simulink model "Pokus02_3bit_Counter"  (Simulink 8.1)
settings: Solver=ode45  StartTime=0.0  StopTime=20  RelTol=1e-3
undefined symbols (not defined in the file): sigbuilder_block
libraries: simulink_extras x17, Common_Library x9, commutil2 x4
settings Model: Creator=uzivatel  LastModifiedBy=uzivatel
settings DataIOCC: SignalLoggingSaveFormat=Dataset
settings OptimizationCC: ExpressionDepthLimit=128
settings DebuggingCC: FcnCallInpInsideContextMsg=EnableAllAsError
settings GRTTargetCC: CombineOutputUpdateFcns=on  GRTInterface=off

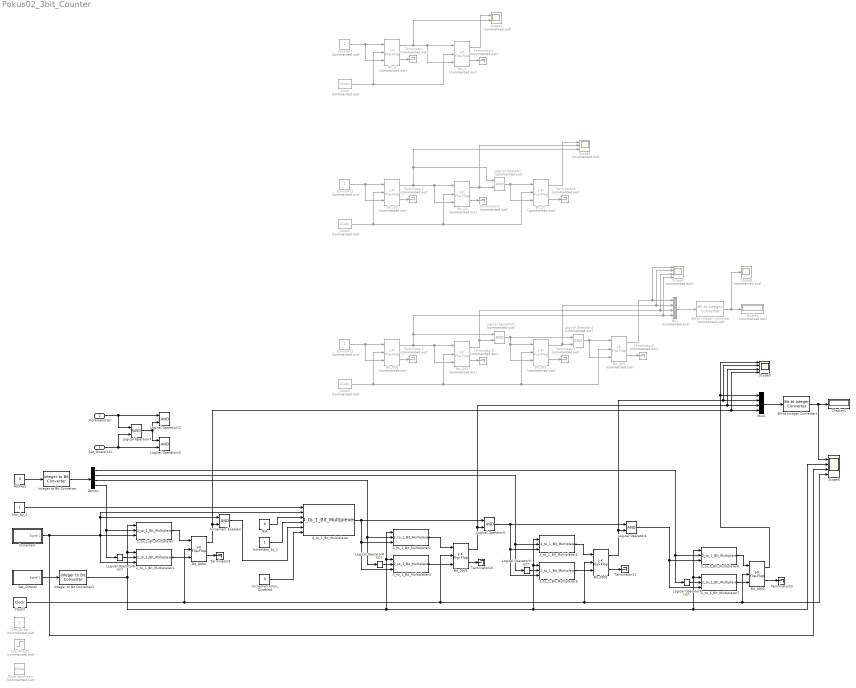
== system Pokus02_3bit_Counter ==
  Set_Direct(1b) : Inport
  Increment(1b) : Inport  Port=2
  2_to_1_Bit_Multiplexer{,1..7} (8 alike) : Common_Library/Multiplexers/2_to_1_Bit_Multiplexer
  4_to_1_Bit_Multiplexer : Common_Library/Multiplexers/4_to_1_Bit_Multiplexer
  Address : Constant  Value=3  OutDataTypeStr=uint8
  Bit to Integer Converter : commutil2/Bit to Integer Converter  Commented=on  nbits=4  bitOrder=MSB first  signedOutputValues=Unsigned  outDtype=uint8  outDtypeSigned=Inherit via internal rule
  Bit to Integer Converter1 : commutil2/Bit to Integer Converter  nbits=4  bitOrder=MSB first  signedOutputValues=Unsigned  outDtype=uint8  outDtypeSigned=Inherit via internal rule
  Bit_0 : simulink_extras/Flip Flops/J-K Flip-Flop  Commented=on  initial_condition=0
  Bit_00 : simulink_extras/Flip Flops/J-K Flip-Flop  Commented=on  initial_condition=0
  Bit_000 : simulink_extras/Flip Flops/J-K Flip-Flop  Commented=on  initial_condition=0
  Bit_0000 : simulink_extras/Flip Flops/J-K Flip-Flop  initial_condition=0
  Bit_0001 : simulink_extras/Flip Flops/J-K Flip-Flop  initial_condition=0
  Bit_0002 : simulink_extras/Flip Flops/J-K Flip-Flop  initial_condition=0
  Bit_0003 : simulink_extras/Flip Flops/J-K Flip-Flop  initial_condition=0
  Bit_001 : simulink_extras/Flip Flops/J-K Flip-Flop  Commented=on  initial_condition=0
  Bit_002 : simulink_extras/Flip Flops/J-K Flip-Flop  Commented=on  initial_condition=0
  Bit_003 : simulink_extras/Flip Flops/J-K Flip-Flop  Commented=on  initial_condition=0
  Bit_01 : simulink_extras/Flip Flops/J-K Flip-Flop  Commented=on  initial_condition=0
  Bit_02 : simulink_extras/Flip Flops/J-K Flip-Flop  Commented=on  initial_condition=0
  Bit_1 : simulink_extras/Flip Flops/J-K Flip-Flop  Commented=on  initial_condition=0
  Clock : simulink_extras/Flip Flops/Clock  Commented=on  period=1
  Clock1 : simulink_extras/Flip Flops/Clock  Commented=on  period=1
  Clock2 : simulink_extras/Flip Flops/Clock  Commented=on  period=1
  Clock3 : simulink_extras/Flip Flops/Clock  period=1
  Constant : Constant  Commented=on  OutDataTypeStr=boolean
  Constant1 : Constant  Commented=on  OutDataTypeStr=boolean
  Constant2 : Constant  Commented=on  OutDataTypeStr=boolean
  Demux : Demux
  Display : Display  Commented=on
  Display1 : Display
  Incr_by_2 : Constant  OutDataTypeStr=boolean
  Increment : Subsystem  Tag=STV Subsys  LoadFcn=sigbuilder_block('load');  StartFcn=sigbuilder_block('start');  StopFcn=sigbuilder_block('stop');  ClipboardFcn=sigbuilder_block('clipboard');  mask(Sigbuilder block){}
      mask help: Simulink:masks:SigbuilderBlock_MD
      mask init:
      | if ~strcmp(get_param(bdroot(gcbh),'SimulationStatus'),'stopped') tuvar = sigbuilder_block('maskInit'); end
      settings: CopyFcn=sigbuilder_block('copy');  DeleteFcn=sigbuilder_block('delete');  ModelCloseFcn=sigbuilder_block('modelClose');  PreSaveFcn=sigbuilder_block('preSave');  PauseFcn=sigbuilder_block('pause');  ContinueFcn=sigbuilder_block('continue');  NameChangeFcn=sigbuilder_block('namechange');  OpenFcn=sigbuilder_block('open',[270 27.75 550.5 399.75 ]);  CloseFcn=sigbuilder_block('close');
      mask Display: plot(0, 0, 100, 100,[2, 2, 32, 32, 2], [68, 8, 8, 68, 68],[32, 2], [38, 38], [32, 19, 2],[53, 60, 44], [32, 17, 17, 2],[16, 16, 31, 31]);txt = getActiveGroup(gcbh);text(2, 100, txt,'verticalAlignment', 'top');
  Increment Enabled : Logic  IconShape=distinctive  AllPortsSameDT=off  OutDataTypeStr=boolean
  Increment_by_2 : Constant  OutDataTypeStr=boolean
  Incrementation_Disabled : Constant  Value=0  OutDataTypeStr=boolean
  Integer to Bit Converter : commutil2/Integer to Bit Converter  nbits=4  signedInputValues=Unsigned  bitOrder=MSB first  outDtype=boolean
  Integer to Bit Converter1 : commutil2/Integer to Bit Converter  nbits=1  signedInputValues=Unsigned  bitOrder=MSB first  outDtype=boolean
  Logical Operator : Logic  Commented=on  IconShape=distinctive  AllPortsSameDT=off  OutDataTypeStr=boolean
  Logical Operator1 : Logic  Commented=on  IconShape=distinctive  AllPortsSameDT=off  OutDataTypeStr=boolean
  Logical Operator{3..4,10..11} (4 alike) : Logic  IconShape=distinctive  AllPortsSameDT=off  OutDataTypeStr=boolean
  Logical Operator2 : Logic  Commented=on  IconShape=distinctive  AllPortsSameDT=off  OutDataTypeStr=boolean
  Logical Operator{5..6,8..9} (4 alike) : Logic  Operator=NOT  IconShape=distinctive  AllPortsSameDT=off  OutDataTypeStr=boolean
  Logical Operator7 : Logic  Operator=NAND  IconShape=distinctive  AllPortsSameDT=off  OutDataTypeStr=boolean
  Mux : Mux  Commented=on
  Mux1 : Mux
  N/A : Constant  Value=0  OutDataTypeStr=boolean
  Pulse Generator : DiscretePulseGenerator  Commented=on  PulseType=Time based  Period=10  PulseWidth=5
  Scope1 : Scope  Commented=on  NumInputPorts=2
      settings: YMin=0~0  YMax=1.5~1.5
  Scope2 : Scope  Commented=on  NumInputPorts=3
      settings: YMin=0~0~0  YMax=1.5~1.5~1.5
  Scope3 : Scope  Commented=on  NumInputPorts=4
      settings: YMin=0~0~0~0  YMax=1.5~1.5~1.5~1.5  SaveName=ScopeData2
  Scope4 : Scope  Commented=on
      settings: YMin=0  YMax=20  SaveName=ScopeData3
  Scope5 : Scope  NumInputPorts=4
      settings: YMin=0~0~0~0  YMax=1.5~1.5~1.5~1.5  SaveName=ScopeData4
  Scope6 : Scope  NumInputPorts=4
      settings: YMin=0~0~0~0  YMax=17~1.5~1.5~1.5  SaveName=ScopeData5
  Set_Direct : Constant  Commented=on  OutDataTypeStr=boolean
  Set_Direct1 : Step  Commented=on  Time=10  SampleTime=0
  Set_Direct2 : Subsystem  Tag=STV Subsys  LoadFcn=sigbuilder_block('load');  StartFcn=sigbuilder_block('start');  StopFcn=sigbuilder_block('stop');  ClipboardFcn=sigbuilder_block('clipboard');  mask(Sigbuilder block){}
      mask help: Simulink:masks:SigbuilderBlock_MD
      mask init:
      | if ~strcmp(get_param(bdroot(gcbh),'SimulationStatus'),'stopped') tuvar = sigbuilder_block('maskInit'); end
      settings: CopyFcn=sigbuilder_block('copy');  DeleteFcn=sigbuilder_block('delete');  ModelCloseFcn=sigbuilder_block('modelClose');  PreSaveFcn=sigbuilder_block('preSave');  PauseFcn=sigbuilder_block('pause');  ContinueFcn=sigbuilder_block('continue');  NameChangeFcn=sigbuilder_block('namechange');  OpenFcn=sigbuilder_block('open',[270 27.75 550.5 399.75 ]);  CloseFcn=sigbuilder_block('close');
      mask Display: plot(0, 0, 100, 100,[2, 2, 32, 32, 2], [68, 8, 8, 68, 68],[32, 2], [38, 38], [32, 19, 2],[53, 60, 44], [32, 17, 17, 2],[16, 16, 31, 31]);txt = getActiveGroup(gcbh);text(2, 100, txt,'verticalAlignment', 'top');
  Terminator{,1..8} (9 alike) : Terminator  Commented=on
  Terminator{9..12} (4 alike) : Terminator
  wires:
  Bit_0/1 -> Bit_1/3, Bit_1/1, Scope1/2
  Constant/1 -> Bit_0/3, Bit_0/1
  Bit_0/2 -> Terminator/1
  Bit_1/2 -> Terminator1/1
  Clock/1 -> Bit_1/2, Bit_0/2
  Bit_1/1 -> Scope1/1
  Constant1/1 -> Bit_00/3, Bit_00/1
  Bit_00/2 -> Terminator2/1
  Bit_01/2 -> Terminator3/1
  Clock1/1 -> Bit_02/2, Bit_01/2, Bit_00/2
  Bit_02/2 -> Terminator4/1
  Bit_02/1 -> Scope2/1
  Bit_00/1 -> Bit_01/3, Bit_01/1, Logical Operator/1, Scope2/3
  Bit_01/1 -> Scope2/2, Logical Operator/2
  Logical Operator/1 -> Bit_02/3, Bit_02/1
  Constant2/1 -> Bit_000/3, Bit_000/1
  Bit_000/2 -> Terminator5/1
  Bit_001/2 -> Terminator6/1
  Clock2/1 -> Bit_003/2, Bit_002/2, Bit_001/2, Bit_000/2
  Bit_002/2 -> Terminator7/1
  Bit_000/1 -> Bit_001/3, Bit_001/1, Scope3/4, Mux/4, Logical Operator1/1
  Bit_001/1 -> Scope3/3, Mux/3, Logical Operator1/2
  Logical Operator1/1 -> Bit_002/3, Bit_002/1, Logical Operator2/1
  Bit_003/2 -> Terminator8/1
  Logical Operator2/1 -> Bit_003/3, Bit_003/1
  Bit_002/1 -> Scope3/2, Mux/2, Logical Operator2/2
  Bit_003/1 -> Scope3/1, Mux/1
  Bit to Integer Converter/1 -> Scope4/1, Display/1
  Mux/1 -> Bit to Integer Converter/1
  Increment/1(Signal 1) -> Scope6/3, 2_to_1_Bit_Multiplexer1/3, 2_to_1_Bit_Multiplexer/3, 4_to_1_Bit_Multiplexer/2, Increment Enabled/1
  Bit_0000/2 -> Terminator9/1
  Bit_0001/2 -> Terminator10/1
  Clock3/1 -> Bit_0000/2, Bit_0002/2, Bit_0003/2, Scope6/4, Bit_0001/2
  Bit_0002/2 -> Terminator11/1
  4_to_1_Bit_Multiplexer/1 -> 2_to_1_Bit_Multiplexer3/3, 2_to_1_Bit_Multiplexer2/3, Logical Operator3/1
  Bit_0001/1 -> Scope5/3, Mux1/3, Logical Operator3/2
  Logical Operator3/1 -> 2_to_1_Bit_Multiplexer5/3, 2_to_1_Bit_Multiplexer4/3, Logical Operator4/1
  Bit_0003/2 -> Terminator12/1
  Logical Operator4/1 -> 2_to_1_Bit_Multiplexer7/3, 2_to_1_Bit_Multiplexer6/3
  Bit_0002/1 -> Scope5/2, Mux1/2, Logical Operator4/2
  Bit_0003/1 -> Scope5/1, Mux1/1
  Bit to Integer Converter1/1 -> Scope6/1, Display1/1
  Mux1/1 -> Bit to Integer Converter1/1
  Address/1 -> Integer to Bit Converter/1
  Demux/4 -> Logical Operator6/1, 2_to_1_Bit_Multiplexer/2
  2_to_1_Bit_Multiplexer1/1 -> Bit_0000/3
  2_to_1_Bit_Multiplexer/1 -> Bit_0000/1
  Logical Operator6/1 -> 2_to_1_Bit_Multiplexer1/2
  Integer to Bit Converter1/1 -> 2_to_1_Bit_Multiplexer/1, 2_to_1_Bit_Multiplexer1/1, 2_to_1_Bit_Multiplexer2/1, 2_to_1_Bit_Multiplexer3/1, 2_to_1_Bit_Multiplexer4/1, 2_to_1_Bit_Multiplexer5/1, 2_to_1_Bit_Multiplexer6/1, 2_to_1_Bit_Multiplexer7/1, Scope6/2
  2_to_1_Bit_Multiplexer2/1 -> Bit_0001/1
  2_to_1_Bit_Multiplexer3/1 -> Bit_0001/3
  Logical Operator8/1 -> 2_to_1_Bit_Multiplexer3/2
  Demux/3 -> Logical Operator8/1, 2_to_1_Bit_Multiplexer2/2
  2_to_1_Bit_Multiplexer4/1 -> Bit_0002/1
  2_to_1_Bit_Multiplexer5/1 -> Bit_0002/3
  Demux/2 -> Logical Operator9/1, 2_to_1_Bit_Multiplexer4/2
  Logical Operator9/1 -> 2_to_1_Bit_Multiplexer5/2
  2_to_1_Bit_Multiplexer7/1 -> Bit_0003/3
  2_to_1_Bit_Multiplexer6/1 -> Bit_0003/1
  Logical Operator5/1 -> 2_to_1_Bit_Multiplexer7/2
  Demux/1 -> Logical Operator5/1, 2_to_1_Bit_Multiplexer6/2
  Integer to Bit Converter/1 -> Demux/1
  Set_Direct2/1(Signal 1) -> Integer to Bit Converter1/1
  Increment(1b)/1 -> Logical Operator11/1, Logical Operator7/1
  Logical Operator7/1 -> Logical Operator11/2, Logical Operator10/1
  Set_Direct(1b)/1 -> Logical Operator7/2, Logical Operator10/2
  Bit_0000/1 -> Scope5/4, Mux1/4, Increment Enabled/2
  N/A/1 -> 4_to_1_Bit_Multiplexer/3
  Incrementation_Disabled/1 -> 4_to_1_Bit_Multiplexer/6
  Increment Enabled/1 -> 4_to_1_Bit_Multiplexer/5
  Increment_by_2/1 -> 4_to_1_Bit_Multiplexer/4
  Incr_by_2/1 -> 4_to_1_Bit_Multiplexer/1

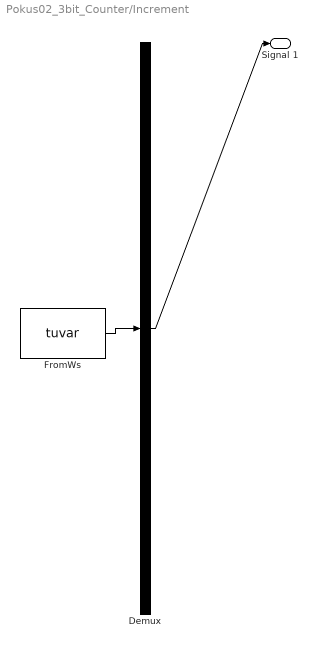
== system Pokus02_3bit_Counter/Increment ==
  Demux : Demux  Tag=STV Demux  Outputs=1
  FromWs : FromWorkspace  Tag=STV FromWs  VariableName=tuvar  SampleTime=0  SigBuilderData=DataTag0  VnvData=DataTag1
      SigBuilderData=|
      | common.afterFinalStr = 'Extrapolate'
      | common.sampleTime = 0
      | dataSet.timeRange = [0 20]
      | dataSet.name = 'Group 1'
      | sbobj.Groups.Name = 'Group 1'
      | sbobj.Groups.Signals.Name = 'Signal 1'
      | sbobj.Groups.Signals.XData = [0 1 1 14 20]
      | sbobj.Groups.Signals.YData = [1 1 0 0 0]
      | sbobj.Groups.TimeRange = [0 20]
  Signal 1 : Outport  Tag=STV Outport
  wires:
  FromWs/1 -> Demux/1
  Demux/1 -> Signal 1/1

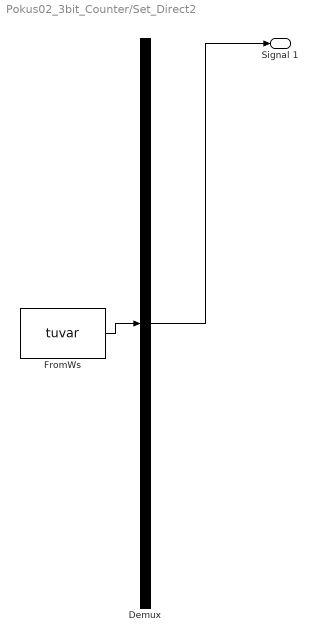
== system Pokus02_3bit_Counter/Set_Direct2 ==
  Demux : Demux  Tag=STV Demux  Outputs=1
  FromWs : FromWorkspace  Tag=STV FromWs  VariableName=tuvar  SampleTime=0  SigBuilderData=DataTag2  VnvData=DataTag3
      SigBuilderData=|
      | common.afterFinalStr = 'Extrapolate'
      | common.sampleTime = 0
      | dataSet.timeRange = [0 20]
      | dataSet.name = 'Group 1'
      | sbobj.Groups.Name = 'Group 1'
      | sbobj.Groups.Signals.Name = 'Signal 1'
      | sbobj.Groups.Signals.XData = [0 13 14 20]
      | sbobj.Groups.Signals.YData = [0 0 0 0]
      | sbobj.Groups.TimeRange = [0 20]
  Signal 1 : Outport  Tag=STV Outport
  wires:
  Demux/1 -> Signal 1/1
  FromWs/1 -> Demux/1
